simulink model "Lookup_nD_verif"  (Simulink 8.4)
settings: Solver=ode45  StartTime=0.0  StopTime=10.0  RelTol=1e-3
undefined symbols (not defined in the file): sigbuilder_block
(part 1 of 2)
settings Model: Creator=Romain  LastModifiedBy=hbourbou
settings DataIOCC: SignalLoggingSaveFormat=Dataset
settings OptimizationCC: ExpressionDepthLimit=128
settings DebuggingCC: SolverPrmCheckMsg=none  FcnCallInpInsideContextMsg=EnableAllAsError  FrameProcessingCompatibilityMsg=error  StateNameClashWarn=none
settings GRTTargetCC: CombineOutputUpdateFcns=on  GRTInterface=off

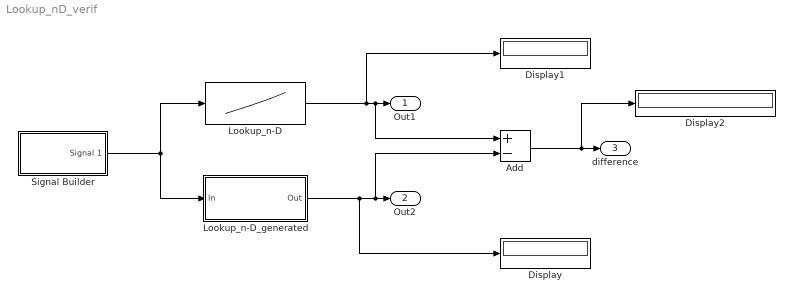
== system Lookup_nD_verif ==
  Add : Sum  Inputs=+-
  Display : Display
  Display1 : Display
  Display2 : Display
  Lookup_n-D : Lookup_n-D  NumberOfTableDimensions=1  BreakpointsForDimension1=[-1.5,-1.4,-1.3,-1.2,-1.1,-1,-0.9,-0.8,-0.7,-0.6,-0.5,-0.4,-0.3,-0.2,-0.1,0,0.1,0.2,0.3,0.4,0.5,0.6,0.7,0.8,0.9,1,1.1,1.2,1.3,1.4,1.5]  Table=[5.42487209386101;6.76686759208599;7.8080705128002;8.69077555288709;9.46124187832334;10.1409773204434;10.7417068159157;11.2704049010402;11.7314396334719;12.1276315881618;12.4608326934196;12.7322661801125;12.9427364629574;13.0927626635598;13.1826640735953;13.2126130786924;13.1826640735953;13.0927626635598;12.9427364629574;12.7322661801125;12.4608326934196;12.1276315881618;11.7314396334719;11.2704049010402;10.7417068159157;10.1409773204434;9.46124187832332;8.6907755528871;7.80807051280015;6.766867592086;5.42487209386099]  RndMeth=Simplest  InputSameDT=on
  Lookup_n-D_generated : Subsystem  TreatAsAtomicUnit=on
  Signal Builder : Subsystem  Tag=STV Subsys  LoadFcn=sigbuilder_block('load');  StartFcn=sigbuilder_block('start');  StopFcn=sigbuilder_block('stop');  ClipboardFcn=sigbuilder_block('clipboard');  mask(Sigbuilder block){}
      mask help: Simulink:masks:SigbuilderBlock_MD
      mask init:
      | if ~strcmp(get_param(bdroot(gcbh),'SimulationStatus'),'stopped') tuvar = sigbuilder_block('maskInit'); end
      settings: CopyFcn=sigbuilder_block('copy');  DeleteFcn=sigbuilder_block('delete');  ModelCloseFcn=sigbuilder_block('modelClose');  PreSaveFcn=sigbuilder_block('preSave');  PauseFcn=sigbuilder_block('pause');  ContinueFcn=sigbuilder_block('continue');  NameChangeFcn=sigbuilder_block('namechange');  OpenFcn=sigbuilder_block('open',[437.6 199.2 550.4 400 ]);  CloseFcn=sigbuilder_block('close');
      mask Display: plot(0, 0, 100, 100,[2, 2, 32, 32, 2], [68, 8, 8, 68, 68],[32, 2], [38, 38], [32, 19, 2],[53, 60, 44], [32, 17, 17, 2],[16, 16, 31, 31]);txt = getActiveGroup(gcbh);text(2, 100, txt,'verticalAlignment', 'top');
  Out1 : Outport
  Out2 : Outport  Port=2
  difference : Outport  Port=3
  wires:
  Signal Builder/1(Signal 1) -> Lookup_n-D_generated/1(In), Lookup_n-D/1
  Lookup_n-D/1 -> Display1/1, Add/1, Out1/1
  Lookup_n-D_generated/1(Out) -> Display/1, Add/2, Out2/1
  Add/1 -> Display2/1, difference/1

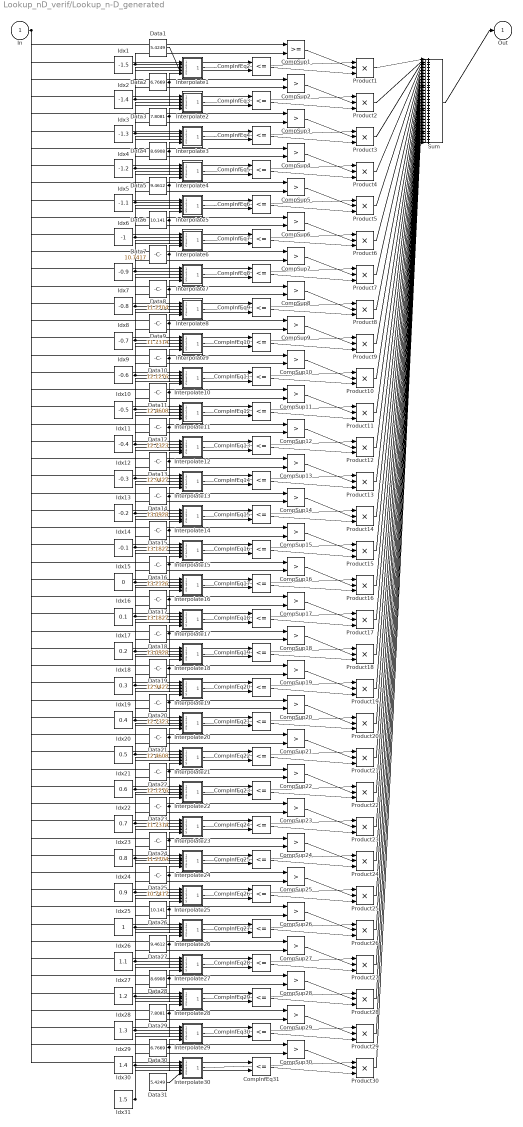
== system Lookup_nD_verif/Lookup_n-D_generated ==
  In : Inport
  CompInfEq{2..31} (30 alike) : RelationalOperator  Operator=<=  InputSameDT=on
  CompSup1 : RelationalOperator  InputSameDT=on
  CompSup{2..30} (29 alike) : RelationalOperator  Operator=>  InputSameDT=on
  Data1 : Constant  Value=5.4249
  Data10 : Constant  Value=12.1276
  Data11 : Constant  Value=12.4608
  Data12 : Constant  Value=12.7323
  Data13 : Constant  Value=12.9427
  Data14 : Constant  Value=13.0928
  Data15 : Constant  Value=13.1827
  Data16 : Constant  Value=13.2126
  Data17 : Constant  Value=13.1827
  Data18 : Constant  Value=13.0928
  Data19 : Constant  Value=12.9427
  Data2 : Constant  Value=6.7669
  Data20 : Constant  Value=12.7323
  Data21 : Constant  Value=12.4608
  Data22 : Constant  Value=12.1276
  Data23 : Constant  Value=11.7314
  Data24 : Constant  Value=11.2704
  Data25 : Constant  Value=10.7417
  Data26 : Constant  Value=10.141
  Data27 : Constant  Value=9.4612
  Data28 : Constant  Value=8.6908
  Data29 : Constant  Value=7.8081
  Data3 : Constant  Value=7.8081
  Data30 : Constant  Value=6.7669
  Data31 : Constant  Value=5.4249
  Data4 : Constant  Value=8.6908
  Data5 : Constant  Value=9.4612
  Data6 : Constant  Value=10.141
  Data7 : Constant  Value=10.7417
  Data8 : Constant  Value=11.2704
  Data9 : Constant  Value=11.7314
  Idx1 : Constant  Value=-1.5
  Idx10 : Constant  Value=-0.6
  Idx11 : Constant  Value=-0.5
  Idx12 : Constant  Value=-0.4
  Idx13 : Constant  Value=-0.3
  Idx14 : Constant  Value=-0.2
  Idx15 : Constant  Value=-0.1
  Idx16 : Constant  Value=0
  Idx17 : Constant  Value=0.1
  Idx18 : Constant  Value=0.2
  Idx19 : Constant  Value=0.3
  Idx2 : Constant  Value=-1.4
  Idx20 : Constant  Value=0.4
  Idx21 : Constant  Value=0.5
  Idx22 : Constant  Value=0.6
  Idx23 : Constant  Value=0.7
  Idx24 : Constant  Value=0.8
  Idx25 : Constant  Value=0.9
  Idx26 : Constant
  Idx27 : Constant  Value=1.1
  Idx28 : Constant  Value=1.2
  Idx29 : Constant  Value=1.3
  Idx3 : Constant  Value=-1.3
  Idx30 : Constant  Value=1.4
  Idx31 : Constant  Value=1.5
  Idx4 : Constant  Value=-1.2
  Idx5 : Constant  Value=-1.1
  Idx6 : Constant  Value=-1
  Idx7 : Constant  Value=-0.9
  Idx8 : Constant  Value=-0.8
  Idx9 : Constant  Value=-0.7
  Interpolate1 : Subsystem  TreatAsAtomicUnit=on
  Interpolate10 : Subsystem  TreatAsAtomicUnit=on
  Interpolate11 : Subsystem  TreatAsAtomicUnit=on
  Interpolate12 : Subsystem  TreatAsAtomicUnit=on
  Interpolate13 : Subsystem  TreatAsAtomicUnit=on
  Interpolate14 : Subsystem  TreatAsAtomicUnit=on
  Interpolate15 : Subsystem  TreatAsAtomicUnit=on
  Interpolate16 : Subsystem  TreatAsAtomicUnit=on
  Interpolate17 : Subsystem  TreatAsAtomicUnit=on
  Interpolate18 : Subsystem  TreatAsAtomicUnit=on
  Interpolate19 : Subsystem  TreatAsAtomicUnit=on
  Interpolate2 : Subsystem  TreatAsAtomicUnit=on
  Interpolate20 : Subsystem  TreatAsAtomicUnit=on
  Interpolate21 : Subsystem  TreatAsAtomicUnit=on
  Interpolate22 : Subsystem  TreatAsAtomicUnit=on
  Interpolate23 : Subsystem  TreatAsAtomicUnit=on
  Interpolate24 : Subsystem  TreatAsAtomicUnit=on
  Interpolate25 : Subsystem  TreatAsAtomicUnit=on
  Interpolate26 : Subsystem  TreatAsAtomicUnit=on
  Interpolate27 : Subsystem  TreatAsAtomicUnit=on
  Interpolate28 : Subsystem  TreatAsAtomicUnit=on
  Interpolate29 : Subsystem  TreatAsAtomicUnit=on
  Interpolate3 : Subsystem  TreatAsAtomicUnit=on
  Interpolate30 : Subsystem  TreatAsAtomicUnit=on
  Interpolate4 : Subsystem  TreatAsAtomicUnit=on
  Interpolate5 : Subsystem  TreatAsAtomicUnit=on
  Interpolate6 : Subsystem  TreatAsAtomicUnit=on
  Interpolate7 : Subsystem  TreatAsAtomicUnit=on
  Interpolate8 : Subsystem  TreatAsAtomicUnit=on
  Interpolate9 : Subsystem  TreatAsAtomicUnit=on
  Product{1..30} (30 alike) : Product  Inputs=***  SaturateOnIntegerOverflow=on  RndMeth=Zero  OutDataTypeStr=Inherit: Same as first input
  Sum : Sum  Inputs=++++++++++++++++++++++++++++++  SaturateOnIntegerOverflow=on  InputSameDT=on  OutDataTypeStr=Inherit: Same as first input
  Out : Outport
  wires:
  In/1 -> Interpolate1/1(InportIn), CompSup1/1, Interpolate2/1(InportIn), CompSup2/1, CompInfEq2/1, Interpolate3/1(InportIn), CompSup3/1, CompInfEq3/1, Interpolate4/1(InportIn), CompSup4/1, CompInfEq4/1, Interpolate5/1(InportIn), CompSup5/1, CompInfEq5/1, Interpolate6/1(InportIn), CompSup6/1, CompInfEq6/1, Interpolate7/1(InportIn), CompSup7/1, CompInfEq7/1, Interpolate8/1(InportIn), CompSup8/1, CompInfEq8/1, Interpolate9/1(InportIn), CompSup9/1, CompInfEq9/1, Interpolate10/1(InportIn), CompSup10/1, CompInfEq10/1, Interpolate11/1(InportIn), CompSup11/1, CompInfEq11/1, Interpolate12/1(InportIn), CompSup12/1, CompInfEq12/1, Interpolate13/1(InportIn), CompSup13/1, CompInfEq13/1, Interpolate14/1(InportIn), CompSup14/1, CompInfEq14/1, Interpolate15/1(InportIn), CompSup15/1, CompInfEq15/1, Interpolate16/1(InportIn), CompSup16/1, CompInfEq16/1, Interpolate17/1(InportIn), CompSup17/1, CompInfEq17/1, Interpolate18/1(InportIn), CompSup18/1, CompInfEq18/1, Interpolate19/1(InportIn), CompSup19/1, CompInfEq19/1, Interpolate20/1(InportIn), CompSup20/1, CompInfEq20/1, Interpolate21/1(InportIn), CompSup21/1, CompInfEq21/1, Interpolate22/1(InportIn), CompSup22/1, CompInfEq22/1, Interpolate23/1(InportIn), CompSup23/1, CompInfEq23/1, Interpolate24/1(InportIn), CompSup24/1, CompInfEq24/1, Interpolate25/1(InportIn), CompSup25/1, CompInfEq25/1, Interpolate26/1(InportIn), CompSup26/1, CompInfEq26/1, Interpolate27/1(InportIn), CompSup27/1, CompInfEq27/1, Interpolate28/1(InportIn), CompSup28/1, CompInfEq28/1, Interpolate29/1(InportIn), CompSup29/1, CompInfEq29/1, Interpolate30/1(InportIn), CompSup30/1, CompInfEq30/1, CompInfEq31/1
  Idx1/1 -> Interpolate1/2(InportIdx1), CompSup1/2
  Data1/1 -> Interpolate1/4(InportData1)
  Interpolate1/1(Out) -> Product1/1
  CompSup1/1 -> Product1/2
  CompInfEq2/1 -> Product1/3
  Product1/1 -> Sum/1
  Idx2/1 -> Interpolate2/2(InportIdx1), CompSup2/2, Interpolate1/3(InportIdx2), CompInfEq2/2
  Data2/1 -> Interpolate2/4(InportData1), Interpolate1/5(InportData2)
  Interpolate2/1(Out) -> Product2/1
  CompSup2/1 -> Product2/2
  CompInfEq3/1 -> Product2/3
  Product2/1 -> Sum/2
  Idx3/1 -> Interpolate3/2(InportIdx1), CompSup3/2, Interpolate2/3(InportIdx2), CompInfEq3/2
  Data3/1 -> Interpolate3/4(InportData1), Interpolate2/5(InportData2)
  Interpolate3/1(Out) -> Product3/1
  CompSup3/1 -> Product3/2
  CompInfEq4/1 -> Product3/3
  Product3/1 -> Sum/3
  Idx4/1 -> Interpolate4/2(InportIdx1), CompSup4/2, Interpolate3/3(InportIdx2), CompInfEq4/2
  Data4/1 -> Interpolate4/4(InportData1), Interpolate3/5(InportData2)
  Interpolate4/1(Out) -> Product4/1
  CompSup4/1 -> Product4/2
  CompInfEq5/1 -> Product4/3
  Product4/1 -> Sum/4
  Idx5/1 -> Interpolate5/2(InportIdx1), CompSup5/2, Interpolate4/3(InportIdx2), CompInfEq5/2
  Data5/1 -> Interpolate5/4(InportData1), Interpolate4/5(InportData2)
  Interpolate5/1(Out) -> Product5/1
  CompSup5/1 -> Product5/2
  CompInfEq6/1 -> Product5/3
  Product5/1 -> Sum/5
  Idx6/1 -> Interpolate6/2(InportIdx1), CompSup6/2, Interpolate5/3(InportIdx2), CompInfEq6/2
  Data6/1 -> Interpolate6/4(InportData1), Interpolate5/5(InportData2)
  Interpolate6/1(Out) -> Product6/1
  CompSup6/1 -> Product6/2
  CompInfEq7/1 -> Product6/3
  Product6/1 -> Sum/6
  Idx7/1 -> Interpolate7/2(InportIdx1), CompSup7/2, Interpolate6/3(InportIdx2), CompInfEq7/2
  Data7/1 -> Interpolate7/4(InportData1), Interpolate6/5(InportData2)
  Interpolate7/1(Out) -> Product7/1
  CompSup7/1 -> Product7/2
  CompInfEq8/1 -> Product7/3
  Product7/1 -> Sum/7
  Idx8/1 -> Interpolate8/2(InportIdx1), CompSup8/2, Interpolate7/3(InportIdx2), CompInfEq8/2
  Data8/1 -> Interpolate8/4(InportData1), Interpolate7/5(InportData2)
  Interpolate8/1(Out) -> Product8/1
  CompSup8/1 -> Product8/2
  CompInfEq9/1 -> Product8/3
  Product8/1 -> Sum/8
  Idx9/1 -> Interpolate9/2(InportIdx1), CompSup9/2, Interpolate8/3(InportIdx2), CompInfEq9/2
  Data9/1 -> Interpolate9/4(InportData1), Interpolate8/5(InportData2)
  Interpolate9/1(Out) -> Product9/1
  CompSup9/1 -> Product9/2
  CompInfEq10/1 -> Product9/3
  Product9/1 -> Sum/9
  Idx10/1 -> Interpolate10/2(InportIdx1), CompSup10/2, Interpolate9/3(InportIdx2), CompInfEq10/2
  Data10/1 -> Interpolate10/4(InportData1), Interpolate9/5(InportData2)
  Interpolate10/1(Out) -> Product10/1
  CompSup10/1 -> Product10/2
  CompInfEq11/1 -> Product10/3
  Product10/1 -> Sum/10
  Idx11/1 -> Interpolate11/2(InportIdx1), CompSup11/2, Interpolate10/3(InportIdx2), CompInfEq11/2
  Data11/1 -> Interpolate11/4(InportData1), Interpolate10/5(InportData2)
  Interpolate11/1(Out) -> Product11/1
  CompSup11/1 -> Product11/2
  CompInfEq12/1 -> Product11/3
  Product11/1 -> Sum/11
  Idx12/1 -> Interpolate12/2(InportIdx1), CompSup12/2, Interpolate11/3(InportIdx2), CompInfEq12/2
  Data12/1 -> Interpolate12/4(InportData1), Interpolate11/5(InportData2)
  Interpolate12/1(Out) -> Product12/1
  CompSup12/1 -> Product12/2
  CompInfEq13/1 -> Product12/3
  Product12/1 -> Sum/12
  Idx13/1 -> Interpolate13/2(InportIdx1), CompSup13/2, Interpolate12/3(InportIdx2), CompInfEq13/2
  Data13/1 -> Interpolate13/4(InportData1), Interpolate12/5(InportData2)
  Interpolate13/1(Out) -> Product13/1
  CompSup13/1 -> Product13/2
  CompInfEq14/1 -> Product13/3
  Product13/1 -> Sum/13
  Idx14/1 -> Interpolate14/2(InportIdx1), CompSup14/2, Interpolate13/3(InportIdx2), CompInfEq14/2
  Data14/1 -> Interpolate14/4(InportData1), Interpolate13/5(InportData2)
  Interpolate14/1(Out) -> Product14/1
  CompSup14/1 -> Product14/2
  CompInfEq15/1 -> Product14/3
  Product14/1 -> Sum/14
  Idx15/1 -> Interpolate15/2(InportIdx1), CompSup15/2, Interpolate14/3(InportIdx2), CompInfEq15/2
  Data15/1 -> Interpolate15/4(InportData1), Interpolate14/5(InportData2)
  Interpolate15/1(Out) -> Product15/1
  CompSup15/1 -> Product15/2
  CompInfEq16/1 -> Product15/3
  Product15/1 -> Sum/15
  Idx16/1 -> Interpolate16/2(InportIdx1), CompSup16/2, Interpolate15/3(InportIdx2), CompInfEq16/2
  Data16/1 -> Interpolate16/4(InportData1), Interpolate15/5(InportData2)
  Interpolate16/1(Out) -> Product16/1
  CompSup16/1 -> Product16/2
  CompInfEq17/1 -> Product16/3
  Product16/1 -> Sum/16
  Idx17/1 -> Interpolate17/2(InportIdx1), CompSup17/2, Interpolate16/3(InportIdx2), CompInfEq17/2
  Data17/1 -> Interpolate17/4(InportData1), Interpolate16/5(InportData2)
  Interpolate17/1(Out) -> Product17/1
  CompSup17/1 -> Product17/2
  CompInfEq18/1 -> Product17/3
  Product17/1 -> Sum/17
  Idx18/1 -> Interpolate18/2(InportIdx1), CompSup18/2, Interpolate17/3(InportIdx2), CompInfEq18/2
  Data18/1 -> Interpolate18/4(InportData1), Interpolate17/5(InportData2)
  Interpolate18/1(Out) -> Product18/1
  CompSup18/1 -> Product18/2
  CompInfEq19/1 -> Product18/3
  Product18/1 -> Sum/18
  Idx19/1 -> Interpolate19/2(InportIdx1), CompSup19/2, Interpolate18/3(InportIdx2), CompInfEq19/2
  Data19/1 -> Interpolate19/4(InportData1), Interpolate18/5(InportData2)
  Interpolate19/1(Out) -> Product19/1
  CompSup19/1 -> Product19/2
  CompInfEq20/1 -> Product19/3
  Product19/1 -> Sum/19
  Idx20/1 -> Interpolate20/2(InportIdx1), CompSup20/2, Interpolate19/3(InportIdx2), CompInfEq20/2
  Data20/1 -> Interpolate20/4(InportData1), Interpolate19/5(InportData2)
  Interpolate20/1(Out) -> Product20/1
  CompSup20/1 -> Product20/2
  CompInfEq21/1 -> Product20/3
  Product20/1 -> Sum/20
  Idx21/1 -> Interpolate21/2(InportIdx1), CompSup21/2, Interpolate20/3(InportIdx2), CompInfEq21/2
  Data21/1 -> Interpolate21/4(InportData1), Interpolate20/5(InportData2)
  Interpolate21/1(Out) -> Product21/1
  CompSup21/1 -> Product21/2
  CompInfEq22/1 -> Product21/3
  Product21/1 -> Sum/21
  Idx22/1 -> Interpolate22/2(InportIdx1), CompSup22/2, Interpolate21/3(InportIdx2), CompInfEq22/2
  Data22/1 -> Interpolate22/4(InportData1), Interpolate21/5(InportData2)
  Interpolate22/1(Out) -> Product22/1
  CompSup22/1 -> Product22/2
  CompInfEq23/1 -> Product22/3
  Product22/1 -> Sum/22
  Idx23/1 -> Interpolate23/2(InportIdx1), CompSup23/2, Interpolate22/3(InportIdx2), CompInfEq23/2
  Data23/1 -> Interpolate23/4(InportData1), Interpolate22/5(InportData2)
  Interpolate23/1(Out) -> Product23/1
  CompSup23/1 -> Product23/2
  CompInfEq24/1 -> Product23/3
  Product23/1 -> Sum/23
  Idx24/1 -> Interpolate24/2(InportIdx1), CompSup24/2, Interpolate23/3(InportIdx2), CompInfEq24/2
  Data24/1 -> Interpolate24/4(InportData1), Interpolate23/5(InportData2)
  Interpolate24/1(Out) -> Product24/1
  CompSup24/1 -> Product24/2
  CompInfEq25/1 -> Product24/3
  Product24/1 -> Sum/24
  Idx25/1 -> Interpolate25/2(InportIdx1), CompSup25/2, Interpolate24/3(InportIdx2), CompInfEq25/2
  Data25/1 -> Interpolate25/4(InportData1), Interpolate24/5(InportData2)
  Interpolate25/1(Out) -> Product25/1
  CompSup25/1 -> Product25/2
  CompInfEq26/1 -> Product25/3
  Product25/1 -> Sum/25
  Idx26/1 -> Interpolate26/2(InportIdx1), CompSup26/2, Interpolate25/3(InportIdx2), CompInfEq26/2
  Data26/1 -> Interpolate26/4(InportData1), Interpolate25/5(InportData2)
  Interpolate26/1(Out) -> Product26/1
  CompSup26/1 -> Product26/2
  CompInfEq27/1 -> Product26/3
  Product26/1 -> Sum/26
  Idx27/1 -> Interpolate27/2(InportIdx1), CompSup27/2, Interpolate26/3(InportIdx2), CompInfEq27/2
  Data27/1 -> Interpolate27/4(InportData1), Interpolate26/5(InportData2)
  Interpolate27/1(Out) -> Product27/1
  CompSup27/1 -> Product27/2
  CompInfEq28/1 -> Product27/3
  Product27/1 -> Sum/27
  Idx28/1 -> Interpolate28/2(InportIdx1), CompSup28/2, Interpolate27/3(InportIdx2), CompInfEq28/2
  Data28/1 -> Interpolate28/4(InportData1), Interpolate27/5(InportData2)
  Interpolate28/1(Out) -> Product28/1
  CompSup28/1 -> Product28/2
  CompInfEq29/1 -> Product28/3
  Product28/1 -> Sum/28
  Idx29/1 -> Interpolate29/2(InportIdx1), CompSup29/2, Interpolate28/3(InportIdx2), CompInfEq29/2
  Data29/1 -> Interpolate29/4(InportData1), Interpolate28/5(InportData2)
  Interpolate29/1(Out) -> Product29/1
  CompSup29/1 -> Product29/2
  CompInfEq30/1 -> Product29/3
  Product29/1 -> Sum/29
  Idx30/1 -> Interpolate30/2(InportIdx1), CompSup30/2, Interpolate29/3(InportIdx2), CompInfEq30/2
  Data30/1 -> Interpolate30/4(InportData1), Interpolate29/5(InportData2)
  Interpolate30/1(Out) -> Product30/1
  CompSup30/1 -> Product30/2
  CompInfEq31/1 -> Product30/3
  Product30/1 -> Sum/30
  Idx31/1 -> Interpolate30/3(InportIdx2), CompInfEq31/2
  Data31/1 -> Interpolate30/5(InportData2)
  Sum/1 -> Out/1

== system Lookup_nD_verif/Signal Builder ==
  Demux : Demux  Tag=STV Demux  Outputs=1
  FromWs : FromWorkspace  Tag=STV FromWs  VariableName=tuvar  SampleTime=0  SigBuilderData=DataTag0  VnvData=DataTag1
      SigBuilderData=|
      | common.afterFinalStr = 'Extrapolate'
      | common.sampleTime = 0
      | dataSet.timeRange = [0 10]
      | dataSet.name = 'Group 1'
      | sbobj.Groups.Name = 'Group 1'
      | sbobj.Groups.Signals.Name = 'Signal 1'
      | sbobj.Groups.Signals.XData = [0 4 4 6 6 10]
      | sbobj.Groups.Signals.YData = [0 0.99 1 0.3 0.26 0]
  Signal 1 : Outport  Tag=STV Outport
  wires:
  Demux/1 -> Signal 1/1
  FromWs/1 -> Demux/1

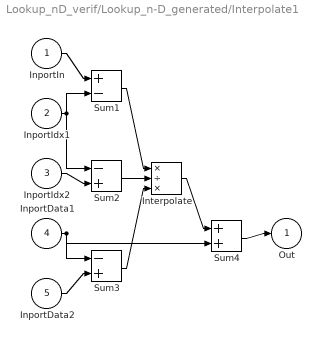
== system Lookup_nD_verif/Lookup_n-D_generated/Interpolate1 ==
  InportIn : Inport
  InportIdx1 : Inport  Port=2
  InportIdx2 : Inport  Port=3
  InportData1 : Inport  Port=4
  InportData2 : Inport  Port=5
  Interpolate : Product  Inputs=*/*  SaturateOnIntegerOverflow=on  RndMeth=Zero  InputSameDT=on  OutDataTypeStr=Inherit: Same as first input
  Sum1 : Sum  Inputs=+-  SaturateOnIntegerOverflow=on  InputSameDT=on  OutDataTypeStr=Inherit: Same as first input
  Sum2 : Sum  Inputs=-+  SaturateOnIntegerOverflow=on  InputSameDT=on  OutDataTypeStr=Inherit: Same as first input
  Sum3 : Sum  Inputs=-+  SaturateOnIntegerOverflow=on  InputSameDT=on  OutDataTypeStr=Inherit: Same as first input
  Sum4 : Sum  SaturateOnIntegerOverflow=on  InputSameDT=on  OutDataTypeStr=Inherit: Same as first input
  Out : Outport
  wires:
  InportIn/1 -> Sum1/1
  InportIdx1/1 -> Sum1/2, Sum2/1
  InportIdx2/1 -> Sum2/2
  InportData1/1 -> Sum3/1, Sum4/2
  InportData2/1 -> Sum3/2
  Sum1/1 -> Interpolate/1
  Sum2/1 -> Interpolate/2
  Sum3/1 -> Interpolate/3
  Interpolate/1 -> Sum4/1
  Sum4/1 -> Out/1

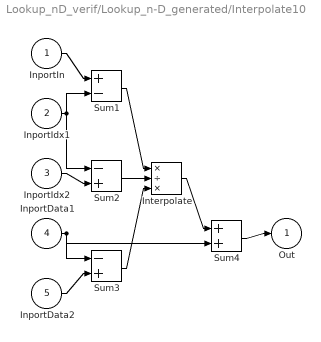
== system Lookup_nD_verif/Lookup_n-D_generated/Interpolate10 ==
  InportIn : Inport
  InportIdx1 : Inport  Port=2
  InportIdx2 : Inport  Port=3
  InportData1 : Inport  Port=4
  InportData2 : Inport  Port=5
  Interpolate : Product  Inputs=*/*  SaturateOnIntegerOverflow=on  RndMeth=Zero  InputSameDT=on  OutDataTypeStr=Inherit: Same as first input
  Sum1 : Sum  Inputs=+-  SaturateOnIntegerOverflow=on  InputSameDT=on  OutDataTypeStr=Inherit: Same as first input
  Sum2 : Sum  Inputs=-+  SaturateOnIntegerOverflow=on  InputSameDT=on  OutDataTypeStr=Inherit: Same as first input
  Sum3 : Sum  Inputs=-+  SaturateOnIntegerOverflow=on  InputSameDT=on  OutDataTypeStr=Inherit: Same as first input
  Sum4 : Sum  SaturateOnIntegerOverflow=on  InputSameDT=on  OutDataTypeStr=Inherit: Same as first input
  Out : Outport
  wires:
  InportIn/1 -> Sum1/1
  InportIdx1/1 -> Sum1/2, Sum2/1
  InportIdx2/1 -> Sum2/2
  InportData1/1 -> Sum3/1, Sum4/2
  InportData2/1 -> Sum3/2
  Sum1/1 -> Interpolate/1
  Sum2/1 -> Interpolate/2
  Sum3/1 -> Interpolate/3
  Interpolate/1 -> Sum4/1
  Sum4/1 -> Out/1

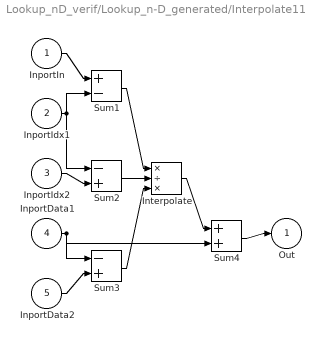
== system Lookup_nD_verif/Lookup_n-D_generated/Interpolate11 ==
  InportIn : Inport
  InportIdx1 : Inport  Port=2
  InportIdx2 : Inport  Port=3
  InportData1 : Inport  Port=4
  InportData2 : Inport  Port=5
  Interpolate : Product  Inputs=*/*  SaturateOnIntegerOverflow=on  RndMeth=Zero  InputSameDT=on  OutDataTypeStr=Inherit: Same as first input
  Sum1 : Sum  Inputs=+-  SaturateOnIntegerOverflow=on  InputSameDT=on  OutDataTypeStr=Inherit: Same as first input
  Sum2 : Sum  Inputs=-+  SaturateOnIntegerOverflow=on  InputSameDT=on  OutDataTypeStr=Inherit: Same as first input
  Sum3 : Sum  Inputs=-+  SaturateOnIntegerOverflow=on  InputSameDT=on  OutDataTypeStr=Inherit: Same as first input
  Sum4 : Sum  SaturateOnIntegerOverflow=on  InputSameDT=on  OutDataTypeStr=Inherit: Same as first input
  Out : Outport
  wires:
  InportIn/1 -> Sum1/1
  InportIdx1/1 -> Sum1/2, Sum2/1
  InportIdx2/1 -> Sum2/2
  InportData1/1 -> Sum3/1, Sum4/2
  InportData2/1 -> Sum3/2
  Sum1/1 -> Interpolate/1
  Sum2/1 -> Interpolate/2
  Sum3/1 -> Interpolate/3
  Interpolate/1 -> Sum4/1
  Sum4/1 -> Out/1

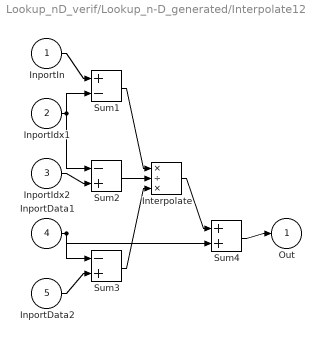
== system Lookup_nD_verif/Lookup_n-D_generated/Interpolate12 ==
  InportIn : Inport
  InportIdx1 : Inport  Port=2
  InportIdx2 : Inport  Port=3
  InportData1 : Inport  Port=4
  InportData2 : Inport  Port=5
  Interpolate : Product  Inputs=*/*  SaturateOnIntegerOverflow=on  RndMeth=Zero  InputSameDT=on  OutDataTypeStr=Inherit: Same as first input
  Sum1 : Sum  Inputs=+-  SaturateOnIntegerOverflow=on  InputSameDT=on  OutDataTypeStr=Inherit: Same as first input
  Sum2 : Sum  Inputs=-+  SaturateOnIntegerOverflow=on  InputSameDT=on  OutDataTypeStr=Inherit: Same as first input
  Sum3 : Sum  Inputs=-+  SaturateOnIntegerOverflow=on  InputSameDT=on  OutDataTypeStr=Inherit: Same as first input
  Sum4 : Sum  SaturateOnIntegerOverflow=on  InputSameDT=on  OutDataTypeStr=Inherit: Same as first input
  Out : Outport
  wires:
  InportIn/1 -> Sum1/1
  InportIdx1/1 -> Sum1/2, Sum2/1
  InportIdx2/1 -> Sum2/2
  InportData1/1 -> Sum3/1, Sum4/2
  InportData2/1 -> Sum3/2
  Sum1/1 -> Interpolate/1
  Sum2/1 -> Interpolate/2
  Sum3/1 -> Interpolate/3
  Interpolate/1 -> Sum4/1
  Sum4/1 -> Out/1

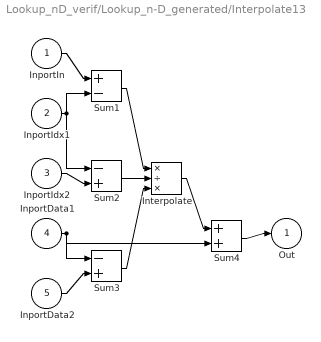
== system Lookup_nD_verif/Lookup_n-D_generated/Interpolate13 ==
  InportIn : Inport
  InportIdx1 : Inport  Port=2
  InportIdx2 : Inport  Port=3
  InportData1 : Inport  Port=4
  InportData2 : Inport  Port=5
  Interpolate : Product  Inputs=*/*  SaturateOnIntegerOverflow=on  RndMeth=Zero  InputSameDT=on  OutDataTypeStr=Inherit: Same as first input
  Sum1 : Sum  Inputs=+-  SaturateOnIntegerOverflow=on  InputSameDT=on  OutDataTypeStr=Inherit: Same as first input
  Sum2 : Sum  Inputs=-+  SaturateOnIntegerOverflow=on  InputSameDT=on  OutDataTypeStr=Inherit: Same as first input
  Sum3 : Sum  Inputs=-+  SaturateOnIntegerOverflow=on  InputSameDT=on  OutDataTypeStr=Inherit: Same as first input
  Sum4 : Sum  SaturateOnIntegerOverflow=on  InputSameDT=on  OutDataTypeStr=Inherit: Same as first input
  Out : Outport
  wires:
  InportIn/1 -> Sum1/1
  InportIdx1/1 -> Sum1/2, Sum2/1
  InportIdx2/1 -> Sum2/2
  InportData1/1 -> Sum3/1, Sum4/2
  InportData2/1 -> Sum3/2
  Sum1/1 -> Interpolate/1
  Sum2/1 -> Interpolate/2
  Sum3/1 -> Interpolate/3
  Interpolate/1 -> Sum4/1
  Sum4/1 -> Out/1

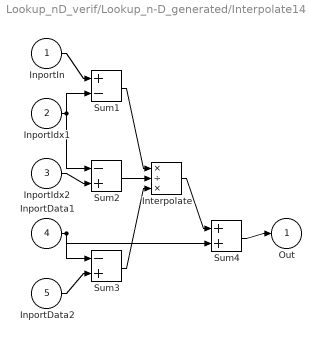
== system Lookup_nD_verif/Lookup_n-D_generated/Interpolate14 ==
  InportIn : Inport
  InportIdx1 : Inport  Port=2
  InportIdx2 : Inport  Port=3
  InportData1 : Inport  Port=4
  InportData2 : Inport  Port=5
  Interpolate : Product  Inputs=*/*  SaturateOnIntegerOverflow=on  RndMeth=Zero  InputSameDT=on  OutDataTypeStr=Inherit: Same as first input
  Sum1 : Sum  Inputs=+-  SaturateOnIntegerOverflow=on  InputSameDT=on  OutDataTypeStr=Inherit: Same as first input
  Sum2 : Sum  Inputs=-+  SaturateOnIntegerOverflow=on  InputSameDT=on  OutDataTypeStr=Inherit: Same as first input
  Sum3 : Sum  Inputs=-+  SaturateOnIntegerOverflow=on  InputSameDT=on  OutDataTypeStr=Inherit: Same as first input
  Sum4 : Sum  SaturateOnIntegerOverflow=on  InputSameDT=on  OutDataTypeStr=Inherit: Same as first input
  Out : Outport
  wires:
  InportIn/1 -> Sum1/1
  InportIdx1/1 -> Sum1/2, Sum2/1
  InportIdx2/1 -> Sum2/2
  InportData1/1 -> Sum3/1, Sum4/2
  InportData2/1 -> Sum3/2
  Sum1/1 -> Interpolate/1
  Sum2/1 -> Interpolate/2
  Sum3/1 -> Interpolate/3
  Interpolate/1 -> Sum4/1
  Sum4/1 -> Out/1

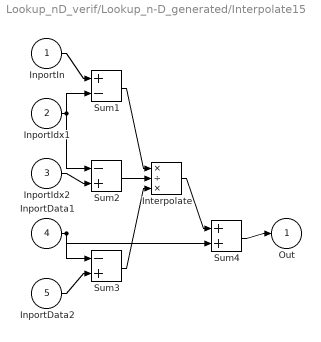
== system Lookup_nD_verif/Lookup_n-D_generated/Interpolate15 ==
  InportIn : Inport
  InportIdx1 : Inport  Port=2
  InportIdx2 : Inport  Port=3
  InportData1 : Inport  Port=4
  InportData2 : Inport  Port=5
  Interpolate : Product  Inputs=*/*  SaturateOnIntegerOverflow=on  RndMeth=Zero  InputSameDT=on  OutDataTypeStr=Inherit: Same as first input
  Sum1 : Sum  Inputs=+-  SaturateOnIntegerOverflow=on  InputSameDT=on  OutDataTypeStr=Inherit: Same as first input
  Sum2 : Sum  Inputs=-+  SaturateOnIntegerOverflow=on  InputSameDT=on  OutDataTypeStr=Inherit: Same as first input
  Sum3 : Sum  Inputs=-+  SaturateOnIntegerOverflow=on  InputSameDT=on  OutDataTypeStr=Inherit: Same as first input
  Sum4 : Sum  SaturateOnIntegerOverflow=on  InputSameDT=on  OutDataTypeStr=Inherit: Same as first input
  Out : Outport
  wires:
  InportIn/1 -> Sum1/1
  InportIdx1/1 -> Sum1/2, Sum2/1
  InportIdx2/1 -> Sum2/2
  InportData1/1 -> Sum3/1, Sum4/2
  InportData2/1 -> Sum3/2
  Sum1/1 -> Interpolate/1
  Sum2/1 -> Interpolate/2
  Sum3/1 -> Interpolate/3
  Interpolate/1 -> Sum4/1
  Sum4/1 -> Out/1

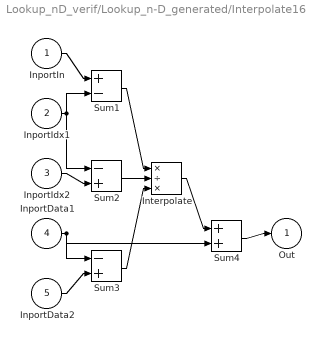
== system Lookup_nD_verif/Lookup_n-D_generated/Interpolate16 ==
  InportIn : Inport
  InportIdx1 : Inport  Port=2
  InportIdx2 : Inport  Port=3
  InportData1 : Inport  Port=4
  InportData2 : Inport  Port=5
  Interpolate : Product  Inputs=*/*  SaturateOnIntegerOverflow=on  RndMeth=Zero  InputSameDT=on  OutDataTypeStr=Inherit: Same as first input
  Sum1 : Sum  Inputs=+-  SaturateOnIntegerOverflow=on  InputSameDT=on  OutDataTypeStr=Inherit: Same as first input
  Sum2 : Sum  Inputs=-+  SaturateOnIntegerOverflow=on  InputSameDT=on  OutDataTypeStr=Inherit: Same as first input
  Sum3 : Sum  Inputs=-+  SaturateOnIntegerOverflow=on  InputSameDT=on  OutDataTypeStr=Inherit: Same as first input
  Sum4 : Sum  SaturateOnIntegerOverflow=on  InputSameDT=on  OutDataTypeStr=Inherit: Same as first input
  Out : Outport
  wires:
  InportIn/1 -> Sum1/1
  InportIdx1/1 -> Sum1/2, Sum2/1
  InportIdx2/1 -> Sum2/2
  InportData1/1 -> Sum3/1, Sum4/2
  InportData2/1 -> Sum3/2
  Sum1/1 -> Interpolate/1
  Sum2/1 -> Interpolate/2
  Sum3/1 -> Interpolate/3
  Interpolate/1 -> Sum4/1
  Sum4/1 -> Out/1

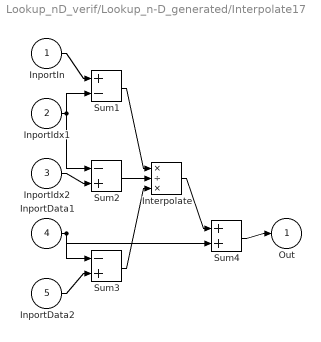
== system Lookup_nD_verif/Lookup_n-D_generated/Interpolate17 ==
  InportIn : Inport
  InportIdx1 : Inport  Port=2
  InportIdx2 : Inport  Port=3
  InportData1 : Inport  Port=4
  InportData2 : Inport  Port=5
  Interpolate : Product  Inputs=*/*  SaturateOnIntegerOverflow=on  RndMeth=Zero  InputSameDT=on  OutDataTypeStr=Inherit: Same as first input
  Sum1 : Sum  Inputs=+-  SaturateOnIntegerOverflow=on  InputSameDT=on  OutDataTypeStr=Inherit: Same as first input
  Sum2 : Sum  Inputs=-+  SaturateOnIntegerOverflow=on  InputSameDT=on  OutDataTypeStr=Inherit: Same as first input
  Sum3 : Sum  Inputs=-+  SaturateOnIntegerOverflow=on  InputSameDT=on  OutDataTypeStr=Inherit: Same as first input
  Sum4 : Sum  SaturateOnIntegerOverflow=on  InputSameDT=on  OutDataTypeStr=Inherit: Same as first input
  Out : Outport
  wires:
  InportIn/1 -> Sum1/1
  InportIdx1/1 -> Sum1/2, Sum2/1
  InportIdx2/1 -> Sum2/2
  InportData1/1 -> Sum3/1, Sum4/2
  InportData2/1 -> Sum3/2
  Sum1/1 -> Interpolate/1
  Sum2/1 -> Interpolate/2
  Sum3/1 -> Interpolate/3
  Interpolate/1 -> Sum4/1
  Sum4/1 -> Out/1

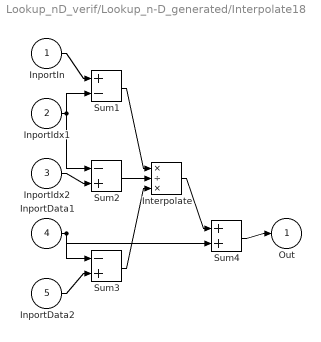
== system Lookup_nD_verif/Lookup_n-D_generated/Interpolate18 ==
  InportIn : Inport
  InportIdx1 : Inport  Port=2
  InportIdx2 : Inport  Port=3
  InportData1 : Inport  Port=4
  InportData2 : Inport  Port=5
  Interpolate : Product  Inputs=*/*  SaturateOnIntegerOverflow=on  RndMeth=Zero  InputSameDT=on  OutDataTypeStr=Inherit: Same as first input
  Sum1 : Sum  Inputs=+-  SaturateOnIntegerOverflow=on  InputSameDT=on  OutDataTypeStr=Inherit: Same as first input
  Sum2 : Sum  Inputs=-+  SaturateOnIntegerOverflow=on  InputSameDT=on  OutDataTypeStr=Inherit: Same as first input
  Sum3 : Sum  Inputs=-+  SaturateOnIntegerOverflow=on  InputSameDT=on  OutDataTypeStr=Inherit: Same as first input
  Sum4 : Sum  SaturateOnIntegerOverflow=on  InputSameDT=on  OutDataTypeStr=Inherit: Same as first input
  Out : Outport
  wires:
  InportIn/1 -> Sum1/1
  InportIdx1/1 -> Sum1/2, Sum2/1
  InportIdx2/1 -> Sum2/2
  InportData1/1 -> Sum3/1, Sum4/2
  InportData2/1 -> Sum3/2
  Sum1/1 -> Interpolate/1
  Sum2/1 -> Interpolate/2
  Sum3/1 -> Interpolate/3
  Interpolate/1 -> Sum4/1
  Sum4/1 -> Out/1

== system Lookup_nD_verif/Lookup_n-D_generated/Interpolate19 ==
  InportIn : Inport
  InportIdx1 : Inport  Port=2
  InportIdx2 : Inport  Port=3
  InportData1 : Inport  Port=4
  InportData2 : Inport  Port=5
  Interpolate : Product  Inputs=*/*  SaturateOnIntegerOverflow=on  RndMeth=Zero  InputSameDT=on  OutDataTypeStr=Inherit: Same as first input
  Sum1 : Sum  Inputs=+-  SaturateOnIntegerOverflow=on  InputSameDT=on  OutDataTypeStr=Inherit: Same as first input
  Sum2 : Sum  Inputs=-+  SaturateOnIntegerOverflow=on  InputSameDT=on  OutDataTypeStr=Inherit: Same as first input
  Sum3 : Sum  Inputs=-+  SaturateOnIntegerOverflow=on  InputSameDT=on  OutDataTypeStr=Inherit: Same as first input
  Sum4 : Sum  SaturateOnIntegerOverflow=on  InputSameDT=on  OutDataTypeStr=Inherit: Same as first input
  Out : Outport
  wires:
  InportIn/1 -> Sum1/1
  InportIdx1/1 -> Sum1/2, Sum2/1
  InportIdx2/1 -> Sum2/2
  InportData1/1 -> Sum3/1, Sum4/2
  InportData2/1 -> Sum3/2
  Sum1/1 -> Interpolate/1
  Sum2/1 -> Interpolate/2
  Sum3/1 -> Interpolate/3
  Interpolate/1 -> Sum4/1
  Sum4/1 -> Out/1

== system Lookup_nD_verif/Lookup_n-D_generated/Interpolate2 ==
  InportIn : Inport
  InportIdx1 : Inport  Port=2
  InportIdx2 : Inport  Port=3
  InportData1 : Inport  Port=4
  InportData2 : Inport  Port=5
  Interpolate : Product  Inputs=*/*  SaturateOnIntegerOverflow=on  RndMeth=Zero  InputSameDT=on  OutDataTypeStr=Inherit: Same as first input
  Sum1 : Sum  Inputs=+-  SaturateOnIntegerOverflow=on  InputSameDT=on  OutDataTypeStr=Inherit: Same as first input
  Sum2 : Sum  Inputs=-+  SaturateOnIntegerOverflow=on  InputSameDT=on  OutDataTypeStr=Inherit: Same as first input
  Sum3 : Sum  Inputs=-+  SaturateOnIntegerOverflow=on  InputSameDT=on  OutDataTypeStr=Inherit: Same as first input
  Sum4 : Sum  SaturateOnIntegerOverflow=on  InputSameDT=on  OutDataTypeStr=Inherit: Same as first input
  Out : Outport
  wires:
  InportIn/1 -> Sum1/1
  InportIdx1/1 -> Sum1/2, Sum2/1
  InportIdx2/1 -> Sum2/2
  InportData1/1 -> Sum3/1, Sum4/2
  InportData2/1 -> Sum3/2
  Sum1/1 -> Interpolate/1
  Sum2/1 -> Interpolate/2
  Sum3/1 -> Interpolate/3
  Interpolate/1 -> Sum4/1
  Sum4/1 -> Out/1

== system Lookup_nD_verif/Lookup_n-D_generated/Interpolate20 ==
  InportIn : Inport
  InportIdx1 : Inport  Port=2
  InportIdx2 : Inport  Port=3
  InportData1 : Inport  Port=4
  InportData2 : Inport  Port=5
  Interpolate : Product  Inputs=*/*  SaturateOnIntegerOverflow=on  RndMeth=Zero  InputSameDT=on  OutDataTypeStr=Inherit: Same as first input
  Sum1 : Sum  Inputs=+-  SaturateOnIntegerOverflow=on  InputSameDT=on  OutDataTypeStr=Inherit: Same as first input
  Sum2 : Sum  Inputs=-+  SaturateOnIntegerOverflow=on  InputSameDT=on  OutDataTypeStr=Inherit: Same as first input
  Sum3 : Sum  Inputs=-+  SaturateOnIntegerOverflow=on  InputSameDT=on  OutDataTypeStr=Inherit: Same as first input
  Sum4 : Sum  SaturateOnIntegerOverflow=on  InputSameDT=on  OutDataTypeStr=Inherit: Same as first input
  Out : Outport
  wires:
  InportIn/1 -> Sum1/1
  InportIdx1/1 -> Sum1/2, Sum2/1
  InportIdx2/1 -> Sum2/2
  InportData1/1 -> Sum3/1, Sum4/2
  InportData2/1 -> Sum3/2
  Sum1/1 -> Interpolate/1
  Sum2/1 -> Interpolate/2
  Sum3/1 -> Interpolate/3
  Interpolate/1 -> Sum4/1
  Sum4/1 -> Out/1

== system Lookup_nD_verif/Lookup_n-D_generated/Interpolate21 ==
  InportIn : Inport
  InportIdx1 : Inport  Port=2
  InportIdx2 : Inport  Port=3
  InportData1 : Inport  Port=4
  InportData2 : Inport  Port=5
  Interpolate : Product  Inputs=*/*  SaturateOnIntegerOverflow=on  RndMeth=Zero  InputSameDT=on  OutDataTypeStr=Inherit: Same as first input
  Sum1 : Sum  Inputs=+-  SaturateOnIntegerOverflow=on  InputSameDT=on  OutDataTypeStr=Inherit: Same as first input
  Sum2 : Sum  Inputs=-+  SaturateOnIntegerOverflow=on  InputSameDT=on  OutDataTypeStr=Inherit: Same as first input
  Sum3 : Sum  Inputs=-+  SaturateOnIntegerOverflow=on  InputSameDT=on  OutDataTypeStr=Inherit: Same as first input
  Sum4 : Sum  SaturateOnIntegerOverflow=on  InputSameDT=on  OutDataTypeStr=Inherit: Same as first input
  Out : Outport
  wires:
  InportIn/1 -> Sum1/1
  InportIdx1/1 -> Sum1/2, Sum2/1
  InportIdx2/1 -> Sum2/2
  InportData1/1 -> Sum3/1, Sum4/2
  InportData2/1 -> Sum3/2
  Sum1/1 -> Interpolate/1
  Sum2/1 -> Interpolate/2
  Sum3/1 -> Interpolate/3
  Interpolate/1 -> Sum4/1
  Sum4/1 -> Out/1

== system Lookup_nD_verif/Lookup_n-D_generated/Interpolate22 ==
  InportIn : Inport
  InportIdx1 : Inport  Port=2
  InportIdx2 : Inport  Port=3
  InportData1 : Inport  Port=4
  InportData2 : Inport  Port=5
  Interpolate : Product  Inputs=*/*  SaturateOnIntegerOverflow=on  RndMeth=Zero  InputSameDT=on  OutDataTypeStr=Inherit: Same as first input
  Sum1 : Sum  Inputs=+-  SaturateOnIntegerOverflow=on  InputSameDT=on  OutDataTypeStr=Inherit: Same as first input
  Sum2 : Sum  Inputs=-+  SaturateOnIntegerOverflow=on  InputSameDT=on  OutDataTypeStr=Inherit: Same as first input
  Sum3 : Sum  Inputs=-+  SaturateOnIntegerOverflow=on  InputSameDT=on  OutDataTypeStr=Inherit: Same as first input
  Sum4 : Sum  SaturateOnIntegerOverflow=on  InputSameDT=on  OutDataTypeStr=Inherit: Same as first input
  Out : Outport
  wires:
  InportIn/1 -> Sum1/1
  InportIdx1/1 -> Sum1/2, Sum2/1
  InportIdx2/1 -> Sum2/2
  InportData1/1 -> Sum3/1, Sum4/2
  InportData2/1 -> Sum3/2
  Sum1/1 -> Interpolate/1
  Sum2/1 -> Interpolate/2
  Sum3/1 -> Interpolate/3
  Interpolate/1 -> Sum4/1
  Sum4/1 -> Out/1

== system Lookup_nD_verif/Lookup_n-D_generated/Interpolate23 ==
  InportIn : Inport
  InportIdx1 : Inport  Port=2
  InportIdx2 : Inport  Port=3
  InportData1 : Inport  Port=4
  InportData2 : Inport  Port=5
  Interpolate : Product  Inputs=*/*  SaturateOnIntegerOverflow=on  RndMeth=Zero  InputSameDT=on  OutDataTypeStr=Inherit: Same as first input
  Sum1 : Sum  Inputs=+-  SaturateOnIntegerOverflow=on  InputSameDT=on  OutDataTypeStr=Inherit: Same as first input
  Sum2 : Sum  Inputs=-+  SaturateOnIntegerOverflow=on  InputSameDT=on  OutDataTypeStr=Inherit: Same as first input
  Sum3 : Sum  Inputs=-+  SaturateOnIntegerOverflow=on  InputSameDT=on  OutDataTypeStr=Inherit: Same as first input
  Sum4 : Sum  SaturateOnIntegerOverflow=on  InputSameDT=on  OutDataTypeStr=Inherit: Same as first input
  Out : Outport
  wires:
  InportIn/1 -> Sum1/1
  InportIdx1/1 -> Sum1/2, Sum2/1
  InportIdx2/1 -> Sum2/2
  InportData1/1 -> Sum3/1, Sum4/2
  InportData2/1 -> Sum3/2
  Sum1/1 -> Interpolate/1
  Sum2/1 -> Interpolate/2
  Sum3/1 -> Interpolate/3
  Interpolate/1 -> Sum4/1
  Sum4/1 -> Out/1

== system Lookup_nD_verif/Lookup_n-D_generated/Interpolate24 ==
  InportIn : Inport
  InportIdx1 : Inport  Port=2
  InportIdx2 : Inport  Port=3
  InportData1 : Inport  Port=4
  InportData2 : Inport  Port=5
  Interpolate : Product  Inputs=*/*  SaturateOnIntegerOverflow=on  RndMeth=Zero  InputSameDT=on  OutDataTypeStr=Inherit: Same as first input
  Sum1 : Sum  Inputs=+-  SaturateOnIntegerOverflow=on  InputSameDT=on  OutDataTypeStr=Inherit: Same as first input
  Sum2 : Sum  Inputs=-+  SaturateOnIntegerOverflow=on  InputSameDT=on  OutDataTypeStr=Inherit: Same as first input
  Sum3 : Sum  Inputs=-+  SaturateOnIntegerOverflow=on  InputSameDT=on  OutDataTypeStr=Inherit: Same as first input
  Sum4 : Sum  SaturateOnIntegerOverflow=on  InputSameDT=on  OutDataTypeStr=Inherit: Same as first input
  Out : Outport
  wires:
  InportIn/1 -> Sum1/1
  InportIdx1/1 -> Sum1/2, Sum2/1
  InportIdx2/1 -> Sum2/2
  InportData1/1 -> Sum3/1, Sum4/2
  InportData2/1 -> Sum3/2
  Sum1/1 -> Interpolate/1
  Sum2/1 -> Interpolate/2
  Sum3/1 -> Interpolate/3
  Interpolate/1 -> Sum4/1
  Sum4/1 -> Out/1

== system Lookup_nD_verif/Lookup_n-D_generated/Interpolate25 ==
  InportIn : Inport
  InportIdx1 : Inport  Port=2
  InportIdx2 : Inport  Port=3
  InportData1 : Inport  Port=4
  InportData2 : Inport  Port=5
  Interpolate : Product  Inputs=*/*  SaturateOnIntegerOverflow=on  RndMeth=Zero  InputSameDT=on  OutDataTypeStr=Inherit: Same as first input
  Sum1 : Sum  Inputs=+-  SaturateOnIntegerOverflow=on  InputSameDT=on  OutDataTypeStr=Inherit: Same as first input
  Sum2 : Sum  Inputs=-+  SaturateOnIntegerOverflow=on  InputSameDT=on  OutDataTypeStr=Inherit: Same as first input
  Sum3 : Sum  Inputs=-+  SaturateOnIntegerOverflow=on  InputSameDT=on  OutDataTypeStr=Inherit: Same as first input
  Sum4 : Sum  SaturateOnIntegerOverflow=on  InputSameDT=on  OutDataTypeStr=Inherit: Same as first input
  Out : Outport
  wires:
  InportIn/1 -> Sum1/1
  InportIdx1/1 -> Sum1/2, Sum2/1
  InportIdx2/1 -> Sum2/2
  InportData1/1 -> Sum3/1, Sum4/2
  InportData2/1 -> Sum3/2
  Sum1/1 -> Interpolate/1
  Sum2/1 -> Interpolate/2
  Sum3/1 -> Interpolate/3
  Interpolate/1 -> Sum4/1
  Sum4/1 -> Out/1

== system Lookup_nD_verif/Lookup_n-D_generated/Interpolate26 ==
  InportIn : Inport
  InportIdx1 : Inport  Port=2
  InportIdx2 : Inport  Port=3
  InportData1 : Inport  Port=4
  InportData2 : Inport  Port=5
  Interpolate : Product  Inputs=*/*  SaturateOnIntegerOverflow=on  RndMeth=Zero  InputSameDT=on  OutDataTypeStr=Inherit: Same as first input
  Sum1 : Sum  Inputs=+-  SaturateOnIntegerOverflow=on  InputSameDT=on  OutDataTypeStr=Inherit: Same as first input
  Sum2 : Sum  Inputs=-+  SaturateOnIntegerOverflow=on  InputSameDT=on  OutDataTypeStr=Inherit: Same as first input
  Sum3 : Sum  Inputs=-+  SaturateOnIntegerOverflow=on  InputSameDT=on  OutDataTypeStr=Inherit: Same as first input
  Sum4 : Sum  SaturateOnIntegerOverflow=on  InputSameDT=on  OutDataTypeStr=Inherit: Same as first input
  Out : Outport
  wires:
  InportIn/1 -> Sum1/1
  InportIdx1/1 -> Sum1/2, Sum2/1
  InportIdx2/1 -> Sum2/2
  InportData1/1 -> Sum3/1, Sum4/2
  InportData2/1 -> Sum3/2
  Sum1/1 -> Interpolate/1
  Sum2/1 -> Interpolate/2
  Sum3/1 -> Interpolate/3
  Interpolate/1 -> Sum4/1
  Sum4/1 -> Out/1

== system Lookup_nD_verif/Lookup_n-D_generated/Interpolate27 ==
  InportIn : Inport
  InportIdx1 : Inport  Port=2
  InportIdx2 : Inport  Port=3
  InportData1 : Inport  Port=4
  InportData2 : Inport  Port=5
  Interpolate : Product  Inputs=*/*  SaturateOnIntegerOverflow=on  RndMeth=Zero  InputSameDT=on  OutDataTypeStr=Inherit: Same as first input
  Sum1 : Sum  Inputs=+-  SaturateOnIntegerOverflow=on  InputSameDT=on  OutDataTypeStr=Inherit: Same as first input
  Sum2 : Sum  Inputs=-+  SaturateOnIntegerOverflow=on  InputSameDT=on  OutDataTypeStr=Inherit: Same as first input
  Sum3 : Sum  Inputs=-+  SaturateOnIntegerOverflow=on  InputSameDT=on  OutDataTypeStr=Inherit: Same as first input
  Sum4 : Sum  SaturateOnIntegerOverflow=on  InputSameDT=on  OutDataTypeStr=Inherit: Same as first input
  Out : Outport
  wires:
  InportIn/1 -> Sum1/1
  InportIdx1/1 -> Sum1/2, Sum2/1
  InportIdx2/1 -> Sum2/2
  InportData1/1 -> Sum3/1, Sum4/2
  InportData2/1 -> Sum3/2
  Sum1/1 -> Interpolate/1
  Sum2/1 -> Interpolate/2
  Sum3/1 -> Interpolate/3
  Interpolate/1 -> Sum4/1
  Sum4/1 -> Out/1

== system Lookup_nD_verif/Lookup_n-D_generated/Interpolate28 ==
  InportIn : Inport
  InportIdx1 : Inport  Port=2
  InportIdx2 : Inport  Port=3
  InportData1 : Inport  Port=4
  InportData2 : Inport  Port=5
  Interpolate : Product  Inputs=*/*  SaturateOnIntegerOverflow=on  RndMeth=Zero  InputSameDT=on  OutDataTypeStr=Inherit: Same as first input
  Sum1 : Sum  Inputs=+-  SaturateOnIntegerOverflow=on  InputSameDT=on  OutDataTypeStr=Inherit: Same as first input
  Sum2 : Sum  Inputs=-+  SaturateOnIntegerOverflow=on  InputSameDT=on  OutDataTypeStr=Inherit: Same as first input
  Sum3 : Sum  Inputs=-+  SaturateOnIntegerOverflow=on  InputSameDT=on  OutDataTypeStr=Inherit: Same as first input
  Sum4 : Sum  SaturateOnIntegerOverflow=on  InputSameDT=on  OutDataTypeStr=Inherit: Same as first input
  Out : Outport
  wires:
  InportIn/1 -> Sum1/1
  InportIdx1/1 -> Sum1/2, Sum2/1
  InportIdx2/1 -> Sum2/2
  InportData1/1 -> Sum3/1, Sum4/2
  InportData2/1 -> Sum3/2
  Sum1/1 -> Interpolate/1
  Sum2/1 -> Interpolate/2
  Sum3/1 -> Interpolate/3
  Interpolate/1 -> Sum4/1
  Sum4/1 -> Out/1

== system Lookup_nD_verif/Lookup_n-D_generated/Interpolate29 ==
  InportIn : Inport
  InportIdx1 : Inport  Port=2
  InportIdx2 : Inport  Port=3
  InportData1 : Inport  Port=4
  InportData2 : Inport  Port=5
  Interpolate : Product  Inputs=*/*  SaturateOnIntegerOverflow=on  RndMeth=Zero  InputSameDT=on  OutDataTypeStr=Inherit: Same as first input
  Sum1 : Sum  Inputs=+-  SaturateOnIntegerOverflow=on  InputSameDT=on  OutDataTypeStr=Inherit: Same as first input
  Sum2 : Sum  Inputs=-+  SaturateOnIntegerOverflow=on  InputSameDT=on  OutDataTypeStr=Inherit: Same as first input
  Sum3 : Sum  Inputs=-+  SaturateOnIntegerOverflow=on  InputSameDT=on  OutDataTypeStr=Inherit: Same as first input
  Sum4 : Sum  SaturateOnIntegerOverflow=on  InputSameDT=on  OutDataTypeStr=Inherit: Same as first input
  Out : Outport
  wires:
  InportIn/1 -> Sum1/1
  InportIdx1/1 -> Sum1/2, Sum2/1
  InportIdx2/1 -> Sum2/2
  InportData1/1 -> Sum3/1, Sum4/2
  InportData2/1 -> Sum3/2
  Sum1/1 -> Interpolate/1
  Sum2/1 -> Interpolate/2
  Sum3/1 -> Interpolate/3
  Interpolate/1 -> Sum4/1
  Sum4/1 -> Out/1

== system Lookup_nD_verif/Lookup_n-D_generated/Interpolate3 ==
  InportIn : Inport
  InportIdx1 : Inport  Port=2
  InportIdx2 : Inport  Port=3
  InportData1 : Inport  Port=4
  InportData2 : Inport  Port=5
  Interpolate : Product  Inputs=*/*  SaturateOnIntegerOverflow=on  RndMeth=Zero  InputSameDT=on  OutDataTypeStr=Inherit: Same as first input
  Sum1 : Sum  Inputs=+-  SaturateOnIntegerOverflow=on  InputSameDT=on  OutDataTypeStr=Inherit: Same as first input
  Sum2 : Sum  Inputs=-+  SaturateOnIntegerOverflow=on  InputSameDT=on  OutDataTypeStr=Inherit: Same as first input
  Sum3 : Sum  Inputs=-+  SaturateOnIntegerOverflow=on  InputSameDT=on  OutDataTypeStr=Inherit: Same as first input
  Sum4 : Sum  SaturateOnIntegerOverflow=on  InputSameDT=on  OutDataTypeStr=Inherit: Same as first input
  Out : Outport
  wires:
  InportIn/1 -> Sum1/1
  InportIdx1/1 -> Sum1/2, Sum2/1
  InportIdx2/1 -> Sum2/2
  InportData1/1 -> Sum3/1, Sum4/2
  InportData2/1 -> Sum3/2
  Sum1/1 -> Interpolate/1
  Sum2/1 -> Interpolate/2
  Sum3/1 -> Interpolate/3
  Interpolate/1 -> Sum4/1
  Sum4/1 -> Out/1

== system Lookup_nD_verif/Lookup_n-D_generated/Interpolate30 ==
  InportIn : Inport
  InportIdx1 : Inport  Port=2
  InportIdx2 : Inport  Port=3
  InportData1 : Inport  Port=4
  InportData2 : Inport  Port=5
  Interpolate : Product  Inputs=*/*  SaturateOnIntegerOverflow=on  RndMeth=Zero  InputSameDT=on  OutDataTypeStr=Inherit: Same as first input
  Sum1 : Sum  Inputs=+-  SaturateOnIntegerOverflow=on  InputSameDT=on  OutDataTypeStr=Inherit: Same as first input
  Sum2 : Sum  Inputs=-+  SaturateOnIntegerOverflow=on  InputSameDT=on  OutDataTypeStr=Inherit: Same as first input
  Sum3 : Sum  Inputs=-+  SaturateOnIntegerOverflow=on  InputSameDT=on  OutDataTypeStr=Inherit: Same as first input
  Sum4 : Sum  SaturateOnIntegerOverflow=on  InputSameDT=on  OutDataTypeStr=Inherit: Same as first input
  Out : Outport
  wires:
  InportIn/1 -> Sum1/1
  InportIdx1/1 -> Sum1/2, Sum2/1
  InportIdx2/1 -> Sum2/2
  InportData1/1 -> Sum3/1, Sum4/2
  InportData2/1 -> Sum3/2
  Sum1/1 -> Interpolate/1
  Sum2/1 -> Interpolate/2
  Sum3/1 -> Interpolate/3
  Interpolate/1 -> Sum4/1
  Sum4/1 -> Out/1

== system Lookup_nD_verif/Lookup_n-D_generated/Interpolate4 ==
  InportIn : Inport
  InportIdx1 : Inport  Port=2
  InportIdx2 : Inport  Port=3
  InportData1 : Inport  Port=4
  InportData2 : Inport  Port=5
  Interpolate : Product  Inputs=*/*  SaturateOnIntegerOverflow=on  RndMeth=Zero  InputSameDT=on  OutDataTypeStr=Inherit: Same as first input
  Sum1 : Sum  Inputs=+-  SaturateOnIntegerOverflow=on  InputSameDT=on  OutDataTypeStr=Inherit: Same as first input
  Sum2 : Sum  Inputs=-+  SaturateOnIntegerOverflow=on  InputSameDT=on  OutDataTypeStr=Inherit: Same as first input
  Sum3 : Sum  Inputs=-+  SaturateOnIntegerOverflow=on  InputSameDT=on  OutDataTypeStr=Inherit: Same as first input
  Sum4 : Sum  SaturateOnIntegerOverflow=on  InputSameDT=on  OutDataTypeStr=Inherit: Same as first input
  Out : Outport
  wires:
  InportIn/1 -> Sum1/1
  InportIdx1/1 -> Sum1/2, Sum2/1
  InportIdx2/1 -> Sum2/2
  InportData1/1 -> Sum3/1, Sum4/2
  InportData2/1 -> Sum3/2
  Sum1/1 -> Interpolate/1
  Sum2/1 -> Interpolate/2
  Sum3/1 -> Interpolate/3
  Interpolate/1 -> Sum4/1
  Sum4/1 -> Out/1

== system Lookup_nD_verif/Lookup_n-D_generated/Interpolate5 ==
  InportIn : Inport
  InportIdx1 : Inport  Port=2
  InportIdx2 : Inport  Port=3
  InportData1 : Inport  Port=4
  InportData2 : Inport  Port=5
  Interpolate : Product  Inputs=*/*  SaturateOnIntegerOverflow=on  RndMeth=Zero  InputSameDT=on  OutDataTypeStr=Inherit: Same as first input
  Sum1 : Sum  Inputs=+-  SaturateOnIntegerOverflow=on  InputSameDT=on  OutDataTypeStr=Inherit: Same as first input
  Sum2 : Sum  Inputs=-+  SaturateOnIntegerOverflow=on  InputSameDT=on  OutDataTypeStr=Inherit: Same as first input
  Sum3 : Sum  Inputs=-+  SaturateOnIntegerOverflow=on  InputSameDT=on  OutDataTypeStr=Inherit: Same as first input
  Sum4 : Sum  SaturateOnIntegerOverflow=on  InputSameDT=on  OutDataTypeStr=Inherit: Same as first input
  Out : Outport
  wires:
  InportIn/1 -> Sum1/1
  InportIdx1/1 -> Sum1/2, Sum2/1
  InportIdx2/1 -> Sum2/2
  InportData1/1 -> Sum3/1, Sum4/2
  InportData2/1 -> Sum3/2
  Sum1/1 -> Interpolate/1
  Sum2/1 -> Interpolate/2
  Sum3/1 -> Interpolate/3
  Interpolate/1 -> Sum4/1
  Sum4/1 -> Out/1

== system Lookup_nD_verif/Lookup_n-D_generated/Interpolate6 ==
  InportIn : Inport
  InportIdx1 : Inport  Port=2
  InportIdx2 : Inport  Port=3
  InportData1 : Inport  Port=4
  InportData2 : Inport  Port=5
  Interpolate : Product  Inputs=*/*  SaturateOnIntegerOverflow=on  RndMeth=Zero  InputSameDT=on  OutDataTypeStr=Inherit: Same as first input
  Sum1 : Sum  Inputs=+-  SaturateOnIntegerOverflow=on  InputSameDT=on  OutDataTypeStr=Inherit: Same as first input
  Sum2 : Sum  Inputs=-+  SaturateOnIntegerOverflow=on  InputSameDT=on  OutDataTypeStr=Inherit: Same as first input
  Sum3 : Sum  Inputs=-+  SaturateOnIntegerOverflow=on  InputSameDT=on  OutDataTypeStr=Inherit: Same as first input
  Sum4 : Sum  SaturateOnIntegerOverflow=on  InputSameDT=on  OutDataTypeStr=Inherit: Same as first input
  Out : Outport
  wires:
  InportIn/1 -> Sum1/1
  InportIdx1/1 -> Sum1/2, Sum2/1
  InportIdx2/1 -> Sum2/2
  InportData1/1 -> Sum3/1, Sum4/2
  InportData2/1 -> Sum3/2
  Sum1/1 -> Interpolate/1
  Sum2/1 -> Interpolate/2
  Sum3/1 -> Interpolate/3
  Interpolate/1 -> Sum4/1
  Sum4/1 -> Out/1

== system Lookup_nD_verif/Lookup_n-D_generated/Interpolate7 ==
  InportIn : Inport
  InportIdx1 : Inport  Port=2
  InportIdx2 : Inport  Port=3
  InportData1 : Inport  Port=4
  InportData2 : Inport  Port=5
  Interpolate : Product  Inputs=*/*  SaturateOnIntegerOverflow=on  RndMeth=Zero  InputSameDT=on  OutDataTypeStr=Inherit: Same as first input
  Sum1 : Sum  Inputs=+-  SaturateOnIntegerOverflow=on  InputSameDT=on  OutDataTypeStr=Inherit: Same as first input
  Sum2 : Sum  Inputs=-+  SaturateOnIntegerOverflow=on  InputSameDT=on  OutDataTypeStr=Inherit: Same as first input
  Sum3 : Sum  Inputs=-+  SaturateOnIntegerOverflow=on  InputSameDT=on  OutDataTypeStr=Inherit: Same as first input
  Sum4 : Sum  SaturateOnIntegerOverflow=on  InputSameDT=on  OutDataTypeStr=Inherit: Same as first input
  Out : Outport
  wires:
  InportIn/1 -> Sum1/1
  InportIdx1/1 -> Sum1/2, Sum2/1
  InportIdx2/1 -> Sum2/2
  InportData1/1 -> Sum3/1, Sum4/2
  InportData2/1 -> Sum3/2
  Sum1/1 -> Interpolate/1
  Sum2/1 -> Interpolate/2
  Sum3/1 -> Interpolate/3
  Interpolate/1 -> Sum4/1
  Sum4/1 -> Out/1

== system Lookup_nD_verif/Lookup_n-D_generated/Interpolate8 ==
  InportIn : Inport
  InportIdx1 : Inport  Port=2
  InportIdx2 : Inport  Port=3
  InportData1 : Inport  Port=4
  InportData2 : Inport  Port=5
  Interpolate : Product  Inputs=*/*  SaturateOnIntegerOverflow=on  RndMeth=Zero  InputSameDT=on  OutDataTypeStr=Inherit: Same as first input
  Sum1 : Sum  Inputs=+-  SaturateOnIntegerOverflow=on  InputSameDT=on  OutDataTypeStr=Inherit: Same as first input
  Sum2 : Sum  Inputs=-+  SaturateOnIntegerOverflow=on  InputSameDT=on  OutDataTypeStr=Inherit: Same as first input
  Sum3 : Sum  Inputs=-+  SaturateOnIntegerOverflow=on  InputSameDT=on  OutDataTypeStr=Inherit: Same as first input
  Sum4 : Sum  SaturateOnIntegerOverflow=on  InputSameDT=on  OutDataTypeStr=Inherit: Same as first input
  Out : Outport
  wires:
  InportIn/1 -> Sum1/1
  InportIdx1/1 -> Sum1/2, Sum2/1
  InportIdx2/1 -> Sum2/2
  InportData1/1 -> Sum3/1, Sum4/2
  InportData2/1 -> Sum3/2
  Sum1/1 -> Interpolate/1
  Sum2/1 -> Interpolate/2
  Sum3/1 -> Interpolate/3
  Interpolate/1 -> Sum4/1
  Sum4/1 -> Out/1
